simulink model "estimate"  (Simulink 5.0)
settings: Solver=ode45  StartTime=0.0  StopTime=10.0  RelTol=1e-3
settings Model: LastModifiedBy=Administrator  BlockReductionOpt=off  BooleanDataType=off

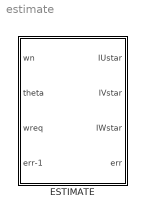
== system estimate ==
  ESTIMATE : Subsystem  mask{N=100, BM=49/60, J=0.0002, DF=0.002, Rr=0.02, Rl=0.03, delta=pi/2, KP=10, KI=5, KD=10, basecurr=34}
      mask prompts: N "Number of turns per phase"; BM "Maximum value of magnetic field intensity"; J "moment of inertia"; DF "viscous friction"; Rr "Rotor radius"; Rl "Rotor length"; delta "phase difference between current nd torque"; KP "Proportionality constant"; KI "Integral constant"; KD "differential constant"; basecurr "rated base current(A)"
      mask help:
      | This block calculates the required calue of current in all the three phases depending upon the speed requirement
      |
      | For good results, phase difference should be kept at pi/2

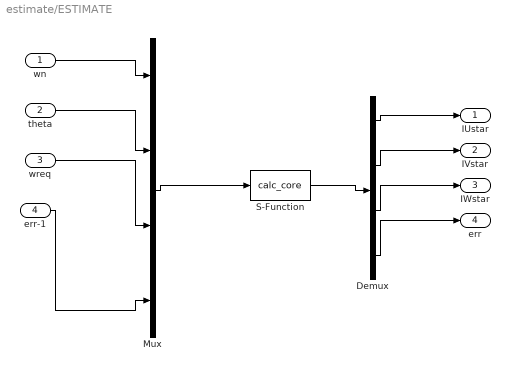
== system estimate/ESTIMATE ==
  wn : Inport
  theta : Inport  Port=2
  wreq : Inport  Port=3
  err-1 : Inport  Port=4
  Demux : Demux
  Mux : Mux
  S-Function : S-Function  FunctionName=calc_core  Parameters=J,DF,N,BM,Rr,Rl,delta,KP,KI,KD,basecurr
  IUstar : Outport
  IVstar : Outport  Port=2
  IWstar : Outport  Port=3
  err : Outport  Port=4
  wires:
  S-Function/1 -> Demux/1
  Mux/1 -> S-Function/1
  err-1/1 -> Mux/4
  wreq/1 -> Mux/3
  theta/1 -> Mux/2
  wn/1 -> Mux/1
  Demux/4 -> err/1
  Demux/3 -> IWstar/1
  Demux/2 -> IVstar/1
  Demux/1 -> IUstar/1
